simulink model "Challenge_Lat_2023_Sim"  (R2023b)
settings: Solver=VariableStepAuto  StartTime=0.0  StopTime=20  RelTol=1e-3
model workspace (MAT data in the model file):
  theta = mpt.Parameter
  theta.Value = 0
  theta.DataType = 'auto'
  theta.Complexity = 'real'
  theta.Dimensions = [1 1]
values from neighbouring files (symbols this model uses):
  a1 = (2*(Caf+Car))/m    (= 65)    [Challenge_Lateral_2023.m]
  a2 = (2*(Caf*lf-Car*lr)/m)    (= -32.75)    [Challenge_Lateral_2023.m]
  a3 = (2*(Caf*lf-Car*lr))/Iz    (= -18.2260869565)    [Challenge_Lateral_2023.m]
  a4 = (2*(Caf*lf^2+Car*lr^2))/Iz    (= 84.6747826087)    [Challenge_Lateral_2023.m]
  Af = 2.2    [Challenge_Lateral_2023.m]    (also in parameters.m)
  b1 = 2*Caf/m    (= 23.75)    [Challenge_Lateral_2023.m]
  b2 = (2*Caf*lf)/Iz    (= 18.5043478261)    [Challenge_Lateral_2023.m]
  Cd = 0.30    (= 0.3)    [Challenge_Lateral_2023.m]    (also in parameters.m)
  Ch = 1-0.085*H    (= 0.9575)    [Challenge_Lateral_2023.m]    (also in parameters.m)
  eta = 0.8    [Challenge_Lateral_2023.m]    (also in parameters.m)
  fr = 0.0328    [Challenge_Lateral_2023.m]    (also in parameters.m)
  g = 9.80665    [Challenge_Lateral_2023.m]    (also in parameters.m)
  m = 1600    [Challenge_Lateral_2023.m]    (also in parameters.m)
  R = 0.30578    [Challenge_Lateral_2023.m]    (also in parameters.m)
  rho = 1.2256    [Challenge_Lateral_2023.m]    (also in parameters.m)
  theta = H/L    (= 0.05)    [Challenge_Lateral_2023.m]    (also in parameters.m)
  Vx_des = 11.12    [Challenge_Lateral_2023.m]    (also in parameters.m)
  y_des = 3    [Challenge_Lateral_2023.m]    (also in parameters.m)
libraries: slpidlib x2
settings Model: Creator=HP  LastModifiedBy=HP

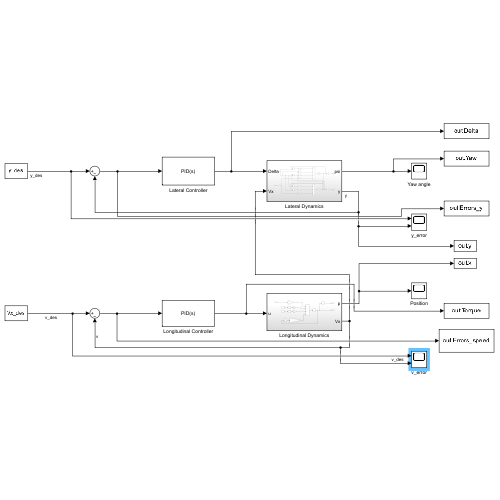
[thumbnail: Simulink's stored preview of the top-level diagram]
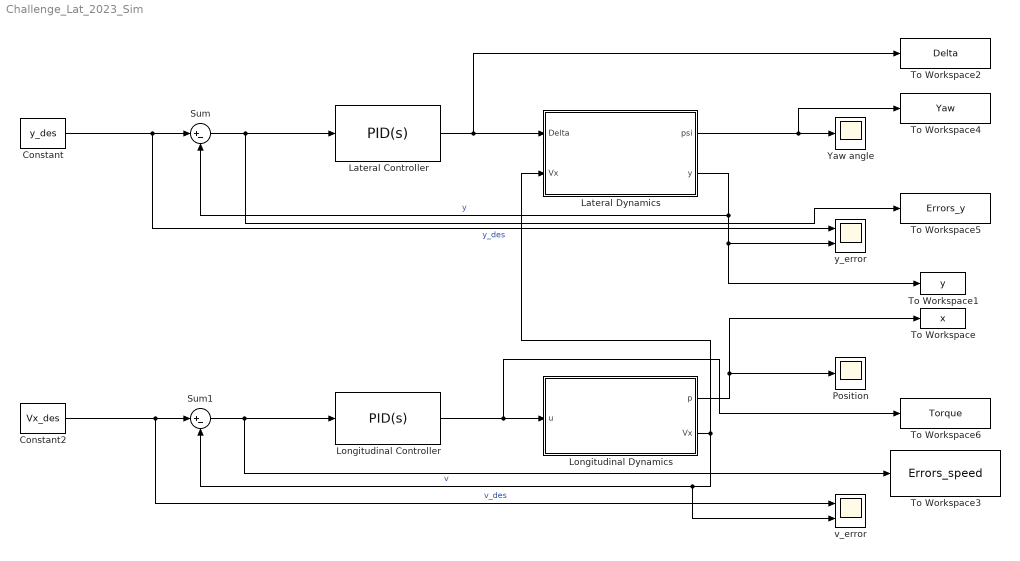
== system Challenge_Lat_2023_Sim ==
  Constant : Constant  Value=y_des
  Constant2 : Constant  Value=Vx_des
  Lateral Controller : slpidlib/PID Controller  Controller=PID  Form=Parallel  TimeDomain=Continuous-time  UseExternalTs=off  SampleTime=-1  IntegratorMethod=Forward Euler  FilterMethod=Forward Euler  ControllerParametersSource=internal  P=1.75  I=0  UseKiTs=off  D=0  N=100  UseFilter=on  TunerSelectOption=Frequency Response Based  InitialConditionSource=internal  InitialConditionForIntegrator=0  InitialConditionForFilter=0  DifferentiatorICPrevScaledInput=0  ExternalReset=none  TrackingMode=off  Kt=1  LimitOutput=off  SatLimitsSource=internal  UpperSaturationLimit=inf  LowerSaturationLimit=-inf  LinearizeAsGain=on  AntiWindupMode=none  Kb=1  LimitIntegrator=off  UpperIntegratorSaturationLimit=inf  LowerIntegratorSaturationLimit=-inf  RndMeth=Zero  POutMin=[]  POutMax=[]  IOutMin=[]  IOutMax=[]  DOutMin=[]  DOutMax=[]  NOutMin=[]  NOutMax=[]  SumOutMin=[]  SumOutMax=[]  SaturationOutMin=[]  SaturationOutMax=[]  PParamMin=[]  PParamMax=[]  IParamMin=[]  IParamMax=[]  DParamMin=[]  DParamMax=[]  NParamMin=[]  NParamMax=[]  KbParamMin=[]  KbParamMax=[]  KtParamMin=[]  KtParamMax=[]  KbOutMin=[]  KbOutMax=[]  KtOutMin=[]  KtOutMax=[]  IntegratorOutMin=[]  IntegratorOutMax=[]  FilterOutMin=[]  FilterOutMax=[]  SumI1OutMin=[]  SumI1OutMax=[]  SumI2OutMin=[]  SumI2OutMax=[]  SumI3OutMin=[]  SumI3OutMax=[]  SumI4OutMin=[]  SumI4OutMax=[]  SumDOutMin=[]  SumDOutMax=[]  DifferentiatorOutMin=[]  DifferentiatorOutMax=[]  FilterDiffOutCoefMin=[]  FilterDiffOutCoefMax=[]  ReciprocalOutMin=[]  ReciprocalOutMax=[]  SumDenOutMin=[]  SumDenOutMax=[]  SumNumOutMin=[]  SumNumOutMax=[]  DivideOutMin=[]  DivideOutMax=[]  UdiffTsProdOutMin=[]  UdiffTsProdOutMax=[]  NTsProdOutMin=[]  NTsProdOutMax=[]  UintegralTsProdOutMin=[]  UintegralTsProdOutMax=[]  UngainTsProdOutMin=[]  UngainTsProdOutMax=[]  ClampingZeroOutDataTypeStr=Inherit: Inherit via back propagation  ClampingZeroOutMin=[]  ClampingZeroOutMax=[]  FilterDenConstantOutDataTypeStr=Inherit: Inherit via back propagation  FilterDenConstantOutMin=[]  FilterDenConstantOutMax=[]  PCopyOutDataTypeStr=Inherit: Inherit via back propagation  PCopyOutMin=[]  PCopyOutMax=[]  NCopyOutDataTypeStr=Inherit: Inherit via back propagation  NCopyOutMin=[]  NCopyOutMax=[]  IntegratorContinuousStateAttributes=''  IntegratorStateMustResolveToSignalObject=off  IntegratorRTWStateStorageClass=Auto  FilterContinuousStateAttributes=''  FilterStateMustResolveToSignalObject=off  FilterRTWStateStorageClass=Auto  ParallelPVariant=InternalParameters  IdealPVariant=Disabled  IVariant=InternalParameters  DVariant=InternalParameters  IntegratorVariant=Continuous  SatVariant=Disabled  AWVariant=Passthrough  PCopyVariant=Disabled  TRVariant=Disabled  FdbkBlocksVariant=Forward  IdealPFdbkVariant=Disabled  SatFdbkVariant=Disabled  DerivativeFilterVariant=ContFilter  NVariant=InternalParameters  NCopyVariant=Disabled  FilterICVariant=InternalICsFilter  IntegratorICVariant=InternalICs  ExternalResetVariant=Disabled  TRSumVariant=Passthrough  SumFdbkVariant=Disabled  SumVariant=Sum_PID  TsampFilterVariant=InternalTs  TsampNgainVariant=Passthrough  TsampIntegralVariant=Disabled_SignalSpec  ExternalSaturationOutDataTypeStr=Inherit: Same as second input
  Lateral Dynamics : Subsystem
  Longitudinal Controller : slpidlib/PID Controller  Controller=PID  Form=Parallel  TimeDomain=Continuous-time  UseExternalTs=off  SampleTime=-1  IntegratorMethod=Forward Euler  FilterMethod=Forward Euler  ControllerParametersSource=internal  P=987.5  I=175  UseKiTs=off  D=0  N=100  UseFilter=on  TunerSelectOption=Frequency Response Based  InitialConditionSource=internal  InitialConditionForIntegrator=0  InitialConditionForFilter=0  DifferentiatorICPrevScaledInput=0  ExternalReset=none  TrackingMode=off  Kt=1  LimitOutput=off  SatLimitsSource=internal  UpperSaturationLimit=inf  LowerSaturationLimit=-inf  LinearizeAsGain=on  AntiWindupMode=none  Kb=1  LimitIntegrator=off  UpperIntegratorSaturationLimit=inf  LowerIntegratorSaturationLimit=-inf  POutMin=[]  POutMax=[]  IOutMin=[]  IOutMax=[]  DOutMin=[]  DOutMax=[]  NOutMin=[]  NOutMax=[]  SumOutMin=[]  SumOutMax=[]  SaturationOutMin=[]  SaturationOutMax=[]  PParamMin=[]  PParamMax=[]  IParamMin=[]  IParamMax=[]  DParamMin=[]  DParamMax=[]  NParamMin=[]  NParamMax=[]  KbParamMin=[]  KbParamMax=[]  KtParamMin=[]  KtParamMax=[]  KbOutMin=[]  KbOutMax=[]  KtOutMin=[]  KtOutMax=[]  IntegratorOutMin=[]  IntegratorOutMax=[]  FilterOutMin=[]  FilterOutMax=[]  SumI1OutMin=[]  SumI1OutMax=[]  SumI2OutMin=[]  SumI2OutMax=[]  SumI3OutMin=[]  SumI3OutMax=[]  SumI4OutMin=[]  SumI4OutMax=[]  SumDOutMin=[]  SumDOutMax=[]  DifferentiatorOutMin=[]  DifferentiatorOutMax=[]  FilterDiffOutCoefMin=[]  FilterDiffOutCoefMax=[]  ReciprocalOutMin=[]  ReciprocalOutMax=[]  SumDenOutMin=[]  SumDenOutMax=[]  SumNumOutMin=[]  SumNumOutMax=[]  DivideOutMin=[]  DivideOutMax=[]  UdiffTsProdOutMin=[]  UdiffTsProdOutMax=[]  NTsProdOutMin=[]  NTsProdOutMax=[]  UintegralTsProdOutMin=[]  UintegralTsProdOutMax=[]  UngainTsProdOutMin=[]  UngainTsProdOutMax=[]  ClampingZeroOutDataTypeStr=Inherit: Inherit via back propagation  ClampingZeroOutMin=[]  ClampingZeroOutMax=[]  FilterDenConstantOutDataTypeStr=Inherit: Inherit via back propagation  FilterDenConstantOutMin=[]  FilterDenConstantOutMax=[]  PCopyOutDataTypeStr=Inherit: Inherit via back propagation  PCopyOutMin=[]  PCopyOutMax=[]  NCopyOutDataTypeStr=Inherit: Inherit via back propagation  NCopyOutMin=[]  NCopyOutMax=[]  IntegratorContinuousStateAttributes=''  IntegratorStateMustResolveToSignalObject=off  IntegratorRTWStateStorageClass=Auto  FilterContinuousStateAttributes=''  FilterStateMustResolveToSignalObject=off  FilterRTWStateStorageClass=Auto  ParallelPVariant=InternalParameters  IdealPVariant=Disabled  IVariant=InternalParameters  DVariant=InternalParameters  IntegratorVariant=Continuous  SatVariant=Disabled  AWVariant=Passthrough  PCopyVariant=Disabled  TRVariant=Disabled  FdbkBlocksVariant=Forward  IdealPFdbkVariant=Disabled  SatFdbkVariant=Disabled  DerivativeFilterVariant=ContFilter  NVariant=InternalParameters  NCopyVariant=Disabled  FilterICVariant=InternalICsFilter  IntegratorICVariant=InternalICs  ExternalResetVariant=Disabled  TRSumVariant=Passthrough  SumFdbkVariant=Disabled  SumVariant=Sum_PID  TsampFilterVariant=InternalTs  TsampNgainVariant=Passthrough  TsampIntegralVariant=Disabled_SignalSpec  ExternalSaturationOutDataTypeStr=Inherit: Same as second input
  Longitudinal Dynamics : Subsystem
  Position : Scope
  Sum : Sum  Inputs=|+-
  Sum1 : Sum  Inputs=|+-
  To Workspace : ToWorkspace  VariableName=x  SampleTime=-1
  To Workspace1 : ToWorkspace  VariableName=y  SampleTime=-1
  To Workspace2 : ToWorkspace  VariableName=Delta  SampleTime=-1
  To Workspace3 : ToWorkspace  VariableName=Errors_speed  SaveFormat=Timeseries  SampleTime=-1
  To Workspace4 : ToWorkspace  VariableName=Yaw  SampleTime=-1
  To Workspace5 : ToWorkspace  VariableName=Errors_y  SampleTime=-1
  To Workspace6 : ToWorkspace  VariableName=Torque  SaveFormat=Timeseries  SampleTime=-1
  Yaw angle : Scope
  v_error : Scope  NumInputPorts=2
  y_error : Scope  NumInputPorts=2
  wires:
  Constant/1 -> y_error/1, Sum/1  "y_des"
  Lateral Controller/1 -> To Workspace2/1, Lateral Dynamics/1(Delta)
  Longitudinal Dynamics/2(Vx) -> Lateral Dynamics/2(Vx), v_error/2, Sum1/2  "v"
  Longitudinal Controller/1 -> To Workspace6/1, Longitudinal Dynamics/1(u)
  Sum1/1 -> To Workspace3/1, Longitudinal Controller/1
  Constant2/1 -> v_error/1, Sum1/1  "v_des"
  Longitudinal Dynamics/1(p) -> To Workspace/1, Position/1
  Lateral Dynamics/2(y) -> Sum/2, To Workspace1/1, y_error/2  "y"
  Lateral Dynamics/1(psi) -> To Workspace4/1, Yaw angle/1
  Sum/1 -> To Workspace5/1, Lateral Controller/1

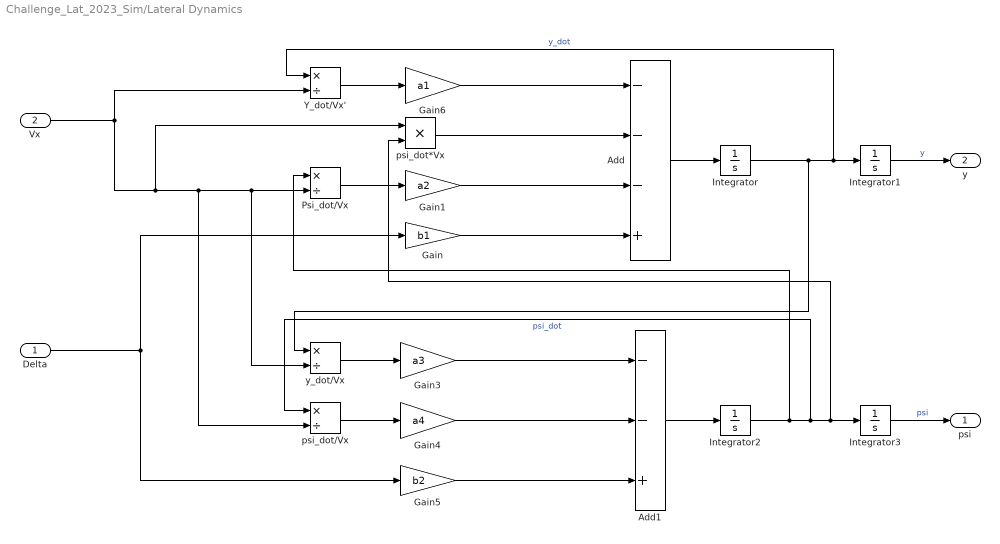
== system Challenge_Lat_2023_Sim/Lateral Dynamics ==
  Delta : Inport
  Vx : Inport  Port=2
  Add : Sum  Inputs=---+
  Add1 : Sum  Inputs=--+
  Gain : Gain  Gain=b1
  Gain1 : Gain  Gain=a2
  Gain3 : Gain  Gain=a3
  Gain4 : Gain  Gain=a4
  Gain5 : Gain  Gain=b2
  Gain6 : Gain  Gain=a1
  Integrator{,1..3} (4 alike) : Integrator
  Psi_dot/Vx : Product  Inputs=*/
  Y_dot/Vx' : Product  Inputs=*/
  psi_dot*Vx : Product
  psi_dot/Vx : Product  Inputs=*/
  y_dot/Vx : Product  Inputs=*/
  psi : Outport
  y : Outport  Port=2
  wires:
  Integrator/1 -> Y_dot/Vx'/1, Integrator1/1, y_dot/Vx/1  "y_dot"
  Integrator3/1 -> psi/1  "psi"
  Add/1 -> Integrator/1
  Integrator2/1 -> Psi_dot/Vx/1, psi_dot/Vx/1, psi_dot*Vx/2, Integrator3/1  "psi_dot"
  Gain3/1 -> Add1/1
  Add1/1 -> Integrator2/1
  Gain5/1 -> Add1/3
  Integrator1/1 -> y/1  "y"
  Gain6/1 -> Add/1
  Gain4/1 -> Add1/2
  Gain1/1 -> Add/3
  Gain/1 -> Add/4
  Delta/1 -> Gain5/1, Gain/1
  Vx/1 -> Psi_dot/Vx/2, y_dot/Vx/2, psi_dot/Vx/2, psi_dot*Vx/1, Y_dot/Vx'/2
  psi_dot*Vx/1 -> Add/2
  Psi_dot/Vx/1 -> Gain1/1
  y_dot/Vx/1 -> Gain3/1
  psi_dot/Vx/1 -> Gain4/1
  Y_dot/Vx'/1 -> Gain6/1

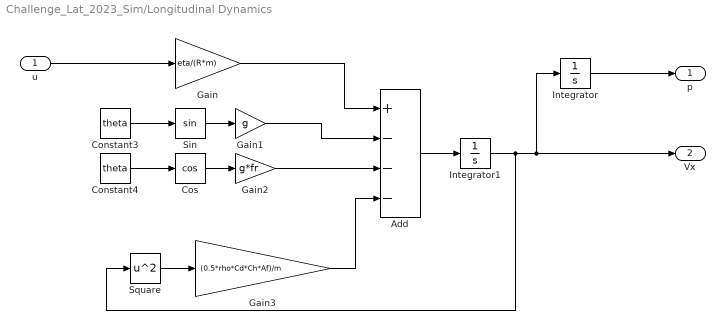
== system Challenge_Lat_2023_Sim/Longitudinal Dynamics ==
  u : Inport
  Add : Sum  Inputs=+---
  Constant3 : Constant  Value=theta
  Constant4 : Constant  Value=theta
  Cos : Trigonometry  Operator=cos
  Gain : Gain  Gain=eta/(R*m)
  Gain1 : Gain  Gain=g
  Gain2 : Gain  Gain=g*fr
  Gain3 : Gain  Gain=(0.5*rho*Cd*Ch*Af)/m
  Integrator : Integrator
  Integrator1 : Integrator  InitialCondition=6.94
  Sin : Trigonometry
  Square : Math  Operator=square
  p : Outport
  Vx : Outport  Port=2
  wires:
  Cos/1 -> Gain2/1
  Gain3/1 -> Add/4
  Gain1/1 -> Add/2
  Gain/1 -> Add/1
  Constant4/1 -> Cos/1
  Constant3/1 -> Sin/1
  Sin/1 -> Gain1/1
  Gain2/1 -> Add/3
  Square/1 -> Gain3/1
  Add/1 -> Integrator1/1
  Integrator1/1 -> Vx/1, Integrator/1, Square/1
  u/1 -> Gain/1
  Integrator/1 -> p/1
